simulink model "lab03"  (R2024a)
settings: Solver=ode4  StartTime=0.0  StopTime=100  FixedStep=0.01  RelTol=1e-3
settings Model: Creator=zv53855  LastModifiedBy=zv53855

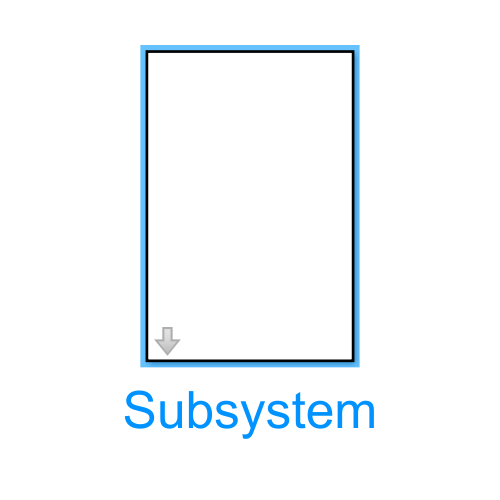
[thumbnail: Simulink's stored preview of the top-level diagram]
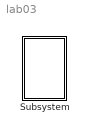
== system lab03 ==
  Subsystem : Subsystem  mask{m=10, k=1, l=3, g=10, phi0=90, phi1=180}

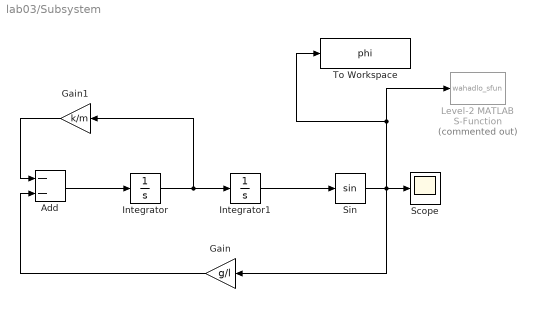
== system lab03/Subsystem ==
  Add : Sum  Inputs=--
  Gain : Gain  Gain=g/l
  Gain1 : Gain  Gain=k/m
  Integrator : Integrator  InitialCondition=phi1*pi/180
  Integrator1 : Integrator  InitialCondition=phi0*pi/180
  Level-2 MATLAB S-Function : M-S-Function  Commented=on  FunctionName=wahadlo_sfun  Parameters=l, m, phi0
  Scope : Scope
  Sin : Trigonometry
  To Workspace : ToWorkspace  VariableName=phi  SampleTime=-1
  wires:
  Gain1/1 -> Add/1
  Sin/1 -> To Workspace/1, Level-2 MATLAB S-Function/1, Gain/1, Scope/1
  Gain/1 -> Add/2
  Add/1 -> Integrator/1
  Integrator1/1 -> Sin/1
  Integrator/1 -> Gain1/1, Integrator1/1
